simulink model "08.half_add"  (R2019b)
settings: Solver=FixedStepAuto  StartTime=0.0  StopTime=inf  FixedStep=1  MaxStep=1  RelTol=1e-3
settings Model: Creator=MARAT  LastModifiedBy=Marat
settings SFSimCC: CustomCodeUndefinedFunction=UseInterfaceOnly

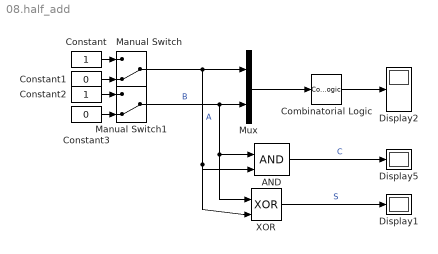
== system 08.half_add ==
  AND : Logic  IconShape=distinctive  AllPortsSameDT=off  OutDataTypeStr=boolean
  Combinatorial Logic : CombinatorialLogic  TruthTable=[0 0; 0 1; 0 1; 1 0]
  Constant : Constant  OutDataTypeStr=boolean
  Constant1 : Constant  Value=0  OutDataTypeStr=boolean
  Constant2 : Constant  OutDataTypeStr=boolean
  Constant3 : Constant  Value=0  OutDataTypeStr=boolean
  Display1 : Display
  Display2 : Display
  Display5 : Display
  Manual Switch : ManualSwitch  CurrentSetting=0
  Manual Switch1 : ManualSwitch  CurrentSetting=0
  Mux : Mux  Inputs=2
  XOR : Logic  Operator=XOR  IconShape=distinctive  AllPortsSameDT=off  OutDataTypeStr=boolean
  wires:
  Mux/1 -> Combinatorial Logic/1
  Combinatorial Logic/1 -> Display2/1
  Constant/1 -> Manual Switch/1
  Constant1/1 -> Manual Switch/2
  Constant3/1 -> Manual Switch1/2
  Constant2/1 -> Manual Switch1/1
  Manual Switch/1 -> XOR/2, AND/2, Mux/1  "A"
  AND/1 -> Display5/1  "C"
  Manual Switch1/1 -> XOR/1, AND/1, Mux/2  "B"
  XOR/1 -> Display1/1  "S"
